simulink model "P702_NI_SoftECU"  (R2019a)
settings: Solver=ode1  StartTime=0.0  StopTime=Inf  FixedStep=0.001  RelTol=1e-3  EnableMultiTasking=on
PreLoadFcn:
  | run '.\VeriStand_BlockSet\NIVeriStandAddPaths.m'
undefined symbols (not defined in the file or in its folder): magnitude
libraries: simulink x83, simulink_extras x1
(part 62 of 76)

== system P702_NI_SoftECU/SoftECU/PCM/Logic1/Key ==
  Bus Creator1 : BusCreator  Inputs=4
  Constant : Constant
  Constant1 : Constant
  Constant2 : Constant
  Constant3 : Constant  Value=3
  Data Type Conversion : DataTypeConversion
  Data Type Conversion1 : DataTypeConversion
  Data Type Conversion2 : DataTypeConversion
  KeyPostn_No : S-Function  Priority=5  FunctionName=NIVeriStandIO  Parameters=width dtype portnum stime stype btype  SFunctionDeploymentMode=off  EnableBusSupport=off  mask(NI VeriStand Inport){portnum=5, width=-1, stime=-1, dtype=auto, stype=auto, btype=1}
      mask prompts: portnum "Port number:"; width "Port dimensions (-1 for dynamically sized):"; stime "Sample time (-1 for inherited):"; dtype "Data type:"; stype "Signal type:"; btype "Block type:"
      mask help: Use this inport on any level of nested subsystems to allow NI VeriStand software to map signals to it.
      mask init:
      | NIVeriStandIO_init;
      settings: CopyFcn=NIVeriStand_MDL_functions('', 'IO_copy');  DeleteFcn=NIVeriStand_MDL_functions('', 'IO_delete');  MoveFcn=set_param(gcb, 'Mask', 'on');
      mask Callback portnum: NIVeriStand_MDL_functions('', 'IO_setportnum');
      mask TypeOptions dtype: auto | double | single | int8 | uint8 | int16 | uint16 | int32 | uint32 | boolean
      mask Callback dtype: NIVeriStand_MDL_functions('', 'IO_booleansignal');
      mask TypeOptions stype: auto | real | complex
      mask Display:
      | patch([-x x], [-y y], [.90980 .81960 .32156]);
      | plot([xrad -x x xrad], [yrad -y y yrad]);
      | fprintf('NI In%d', portnum);
  KeyType_No : Constant
  KvActive : S-Function  Priority=1  FunctionName=NIVeriStandIO  Parameters=width dtype portnum stime stype btype  SFunctionDeploymentMode=off  EnableBusSupport=off  mask(NI VeriStand Inport){portnum=1, width=-1, stime=-1, dtype=auto, stype=auto, btype=1}
      mask prompts: portnum "Port number:"; width "Port dimensions (-1 for dynamically sized):"; stime "Sample time (-1 for inherited):"; dtype "Data type:"; stype "Signal type:"; btype "Block type:"
      mask help: Use this inport on any level of nested subsystems to allow NI VeriStand software to map signals to it.
      mask init:
      | NIVeriStandIO_init;
      settings: CopyFcn=NIVeriStand_MDL_functions('', 'IO_copy');  DeleteFcn=NIVeriStand_MDL_functions('', 'IO_delete');  MoveFcn=set_param(gcb, 'Mask', 'on');
      mask Callback portnum: NIVeriStand_MDL_functions('', 'IO_setportnum');
      mask TypeOptions dtype: auto | double | single | int8 | uint8 | int16 | uint16 | int32 | uint32 | boolean
      mask Callback dtype: NIVeriStand_MDL_functions('', 'IO_booleansignal');
      mask TypeOptions stype: auto | real | complex
      mask Display:
      | patch([-x x], [-y y], [.90980 .81960 .32156]);
      | plot([xrad -x x xrad], [yrad -y y yrad]);
      | fprintf('NI In%d', portnum);
  Logical Operator1 : Logic  Operator=OR  AllPortsSameDT=off  OutDataTypeStr=boolean
  PowerStates : Subsystem
  Start/Stop_Pulsing : Subsystem
  StartBttnPressReq_No : S-Function  Priority=3  FunctionName=NIVeriStandIO  Parameters=width dtype portnum stime stype btype  SFunctionDeploymentMode=off  EnableBusSupport=off  mask(NI VeriStand Inport){portnum=3, width=-1, stime=-1, dtype=auto, stype=auto, btype=1}
      mask prompts: portnum "Port number:"; width "Port dimensions (-1 for dynamically sized):"; stime "Sample time (-1 for inherited):"; dtype "Data type:"; stype "Signal type:"; btype "Block type:"
      mask help: Use this inport on any level of nested subsystems to allow NI VeriStand software to map signals to it.
      mask init:
      | NIVeriStandIO_init;
      settings: CopyFcn=NIVeriStand_MDL_functions('', 'IO_copy');  DeleteFcn=NIVeriStand_MDL_functions('', 'IO_delete');  MoveFcn=set_param(gcb, 'Mask', 'on');
      mask Callback portnum: NIVeriStand_MDL_functions('', 'IO_setportnum');
      mask TypeOptions dtype: auto | double | single | int8 | uint8 | int16 | uint16 | int32 | uint32 | boolean
      mask Callback dtype: NIVeriStand_MDL_functions('', 'IO_booleansignal');
      mask TypeOptions stype: auto | real | complex
      mask Display:
      | patch([-x x], [-y y], [.90980 .81960 .32156]);
      | plot([xrad -x x xrad], [yrad -y y yrad]);
      | fprintf('NI In%d', portnum);
  StartBttnSw1_B : S-Function  Priority=2  FunctionName=NIVeriStandIO  Parameters=width dtype portnum stime stype btype  SFunctionDeploymentMode=off  EnableBusSupport=off  mask(NI VeriStand Inport){portnum=2, width=-1, stime=-1, dtype=auto, stype=auto, btype=1}
      mask prompts: portnum "Port number:"; width "Port dimensions (-1 for dynamically sized):"; stime "Sample time (-1 for inherited):"; dtype "Data type:"; stype "Signal type:"; btype "Block type:"
      mask help: Use this inport on any level of nested subsystems to allow NI VeriStand software to map signals to it.
      mask init:
      | NIVeriStandIO_init;
      settings: CopyFcn=NIVeriStand_MDL_functions('', 'IO_copy');  DeleteFcn=NIVeriStand_MDL_functions('', 'IO_delete');  MoveFcn=set_param(gcb, 'Mask', 'on');
      mask Callback portnum: NIVeriStand_MDL_functions('', 'IO_setportnum');
      mask TypeOptions dtype: auto | double | single | int8 | uint8 | int16 | uint16 | int32 | uint32 | boolean
      mask Callback dtype: NIVeriStand_MDL_functions('', 'IO_booleansignal');
      mask TypeOptions stype: auto | real | complex
      mask Display:
      | patch([-x x], [-y y], [.90980 .81960 .32156]);
      | plot([xrad -x x xrad], [yrad -y y yrad]);
      | fprintf('NI In%d', portnum);
  Switch{,1..3} (4 alike) : Switch  Criteria=u2 > Threshold
  Switch_NI_Port_Pcm : S-Function  Priority=4  FunctionName=NIVeriStandIO  Parameters=width dtype portnum stime stype btype  SFunctionDeploymentMode=off  EnableBusSupport=off  mask(NI VeriStand Inport){portnum=4, width=-1, stime=-1, dtype=auto, stype=auto, btype=1}
      mask prompts: portnum "Port number:"; width "Port dimensions (-1 for dynamically sized):"; stime "Sample time (-1 for inherited):"; dtype "Data type:"; stype "Signal type:"; btype "Block type:"
      mask help: Use this inport on any level of nested subsystems to allow NI VeriStand software to map signals to it.
      mask init:
      | NIVeriStandIO_init;
      settings: CopyFcn=NIVeriStand_MDL_functions('', 'IO_copy');  DeleteFcn=NIVeriStand_MDL_functions('', 'IO_delete');  MoveFcn=set_param(gcb, 'Mask', 'on');
      mask Callback portnum: NIVeriStand_MDL_functions('', 'IO_setportnum');
      mask TypeOptions dtype: auto | double | single | int8 | uint8 | int16 | uint16 | int32 | uint32 | boolean
      mask Callback dtype: NIVeriStand_MDL_functions('', 'IO_booleansignal');
      mask TypeOptions stype: auto | real | complex
      mask Display:
      | patch([-x x], [-y y], [.90980 .81960 .32156]);
      | plot([xrad -x x xrad], [yrad -y y yrad]);
      | fprintf('NI In%d', portnum);
  Out1 : Outport
  wires:
  KeyType_No/1 -> Bus Creator1/2  "KeyType_No"
  Switch3/1 -> PowerStates/1(In1), Bus Creator1/3  "KeyPostn_No"
  Bus Creator1/1 -> Out1/1  "Key"
  PowerStates/1(Out1) -> Bus Creator1/4  "PowerStates"
  Logical Operator1/1 -> PowerStates/2(In2), Bus Creator1/1  "StartBttnSw1_B"
  Start/Stop_Pulsing/1(Out1) -> Logical Operator1/1
  StartBttnSw1_B/1 -> Data Type Conversion1/1
  StartBttnPressReq_No/1 -> Switch/1
  KvActive/1 -> Switch2/1
  Switch/1 -> Start/Stop_Pulsing/1(In1)
  Switch1/1 -> Logical Operator1/2
  Switch2/1 -> PowerStates/3(In3)
  Switch_NI_Port_Pcm/1 -> Data Type Conversion/1
  KeyPostn_No/1 -> Switch3/1
  Constant/1 -> Switch/3
  Constant1/1 -> Data Type Conversion2/1
  Constant2/1 -> Switch2/3
  Constant3/1 -> Switch3/3
  Data Type Conversion/1 -> Switch3/2, Switch2/2, Switch1/2, Switch/2
  Data Type Conversion1/1 -> Switch1/1
  Data Type Conversion2/1 -> Switch1/3

== system P702_NI_SoftECU/SoftECU/PCM/Logic1/Pedals ==
  FromMdl : Inport
  Bias : Bias  Bias=1
  BrakeLight : Constant  Value=0
  Bus Creator : BusCreator  Inputs=7
  Bus Selector : BusSelector  OutputSignals=CluBottomOfTravelSwtch_B,Throttle[percentage],BrkLightSwtch_B
  Constant : Constant  Value=3
  Derivative1 : Derivative
  Derivative2 : Derivative
  Pedals : Outport
  wires:
  Bias/1 -> Bus Creator/3  "BrakePdlDrvAppl"
  FromMdl/1 -> Bus Selector/1
  BrakeLight/1 -> Bias/1
  Derivative2/1 -> Bus Creator/2  "ApedPosRate"
  Bus Selector/2 -> Derivative2/1, Bus Creator/5  "<Throttle[percentage]>"
  Bus Creator/1 -> Pedals/1  "Pedals"
  Bus Selector/1 -> Derivative1/1, Bus Creator/4  "<CluBottomOfTravelSwtch_B>"
  Derivative1/1 -> Bus Creator/1  "CluPdlRate"
  Bus Selector/3 -> Bus Creator/6  "<BrkLightSwtch_B>"
  Constant/1 -> Bus Creator/7  "CluPdlPosPcMeas_D_Qf"

== system P702_NI_SoftECU/SoftECU/PCM/Logic1/PrplWhlTot2Calc ==
  note: R = -1
      | N = 0
      | 1 ... 6 =  1 ... 6
  note: -> Tire Torque
  Gear : Inport
  Trq_Engine [Nm] : Inport  Port=2
  GetTransmissionRatio : Subsystem
      mask Display: disp('Get current transmission ratio')
  Mult : Product  RndMeth=Zero
  PrplWhlTot_Tq : Outport
  wires:
  Gear/1 -> GetTransmissionRatio/1(Gear[-])
  GetTransmissionRatio/1(Transmission_Ratio[-]) -> Mult/2
  Trq_Engine [Nm]/1 -> Mult/1
  Mult/1 -> PrplWhlTot_Tq/1

== system P702_NI_SoftECU/SoftECU/PCM/Logic1/ReValueStates ==
  note: SelectorLever[-3T|-2P|-1R|0N|1D]
  note: GearlvrPosDActl[-1Unknown|0P|1R|2N|3D]
  GearLvr[-] : Inport
  AddOffset_for_R-N_gears : Sum
  OffsetForSw : Constant  Value=2
  Transmission_Ratio[-] : Outport
  wires:
  AddOffset_for_R-N_gears/1 -> Transmission_Ratio[-]/1  "GearLvrPos_D_ActlPart"
  OffsetForSw/1 -> AddOffset_for_R-N_gears/2
  GearLvr[-]/1 -> AddOffset_for_R-N_gears/1

== system P702_NI_SoftECU/SoftECU/PCM/Logic1/Speed_Accel_Controller ==
  note: ACC status = 0:
      | ACC off-> ignore accel and decel control, throttle and brake controlled by speed controller
      | ACC status = 1:
      | ACC ON->ignore speed controller, throttle and brake controller by acceleration controller
      | ver. 10/23/2018 ;
  ACC_Status : Inport
  Veh_Spd : Inport  Port=2
  Desired_Speed : Inport  Port=3
  vehicle_accel : Inport  Port=4
  Desried_accel : Inport  Port=5
  cmbb_rq : Inport  Port=6
  MRR : Inport  Port=7
  ACC_Accel_Controller : Subsystem
  BrakeMSPress_switch : MultiPortSwitch  DataPortOrder=Zero-based contiguous  Inputs=2  zeroidx=on
  Compare To Constant : simulink/Logic and Bit Operations/Compare To Constant  relop===  const=5  OutDataTypeStr=boolean
  Compare To Constant1 : simulink/Logic and Bit Operations/Compare To Constant  relop===  const=4  OutDataTypeStr=boolean
  Ground : Ground
  Logical Operator : Logic  Operator=OR  AllPortsSameDT=off  OutDataTypeStr=boolean
  MATLAB Function : MATLAB Function  TreatAsAtomicUnit=on
  MATLAB Function1 : MATLAB Function  TreatAsAtomicUnit=on
  Speed_Controller : Subsystem
  Terminator : Terminator
  Terminator1 : Terminator
  Terminator3 : Terminator
  throttle_switch : MultiPortSwitch  DataPortOrder=Zero-based contiguous  Inputs=2  zeroidx=on
  throttle_position : Outport
  brake_MS_pressure : Outport  Port=2
  wires:
  Speed_Controller/1(Throttle_Pos) -> MATLAB Function1/1(throttle_pos)
  ACC_Accel_Controller/1(Throttle_Pos) -> throttle_switch/3
  Speed_Controller/2(Brake_MS_Pressure) -> BrakeMSPress_switch/2
  ACC_Accel_Controller/2(Brake_MS_Pressure) -> BrakeMSPress_switch/3
  ACC_Status/1 -> Compare To Constant1/1, Compare To Constant/1
  Veh_Spd/1 -> Terminator/1, Speed_Controller/1(Veh_Spd)
  throttle_switch/1 -> throttle_position/1
  vehicle_accel/1 -> ACC_Accel_Controller/1(Vehicle_Ax)
  Desried_accel/1 -> ACC_Accel_Controller/2(Desried_accel)
  Logical Operator/1 -> BrakeMSPress_switch/1, throttle_switch/1
  BrakeMSPress_switch/1 -> brake_MS_pressure/1
  Compare To Constant/1 -> Logical Operator/1
  Compare To Constant1/1 -> Logical Operator/2
  cmbb_rq/1 -> MATLAB Function1/2(cmbb_req)
  MRR/1 -> Terminator1/1
  Ground/1 -> MATLAB Function/4(mrr), MATLAB Function/3(desired_speed_rq), MATLAB Function/2(cmbb_req), MATLAB Function/1(veh_speed)
  MATLAB Function/1(desired_speed) -> Terminator3/1
  Desired_Speed/1 -> Speed_Controller/2(Desried_Spd)
  MATLAB Function1/1(throttle) -> throttle_switch/2

== system P702_NI_SoftECU/SoftECU/PCM/Logic1/StartStop ==
  Eng_D_Stat : Inport
  Cranking_status : Inport  Port=2
  Compare To Constant : simulink/Logic and Bit Operations/Compare To Constant  relop===  const=1  OutDataTypeStr=uint8
  Logical Operator : Logic  Operator=NOT  AllPortsSameDT=off  OutDataTypeStr=boolean
  Logical Operator1 : Logic  AllPortsSameDT=off  OutDataTypeStr=boolean
  dt_ElPw_D_StatStrtStop : DataTypeConversion  RndMeth=Zero
  StatStrtStop : Outport
  Cranking_status_out : Outport  Port=2
  wires:
  Logical Operator1/1 -> dt_ElPw_D_StatStrtStop/1
  Logical Operator/1 -> Logical Operator1/2
  Compare To Constant/1 -> Logical Operator1/1
  Cranking_status/1 -> Cranking_status_out/1, Logical Operator/1  "PcmCrankingStatus_B"
  dt_ElPw_D_StatStrtStop/1 -> StatStrtStop/1  "StatStrtStop"
  Eng_D_Stat/1 -> Compare To Constant/1  "Eng_D_Stat_No"

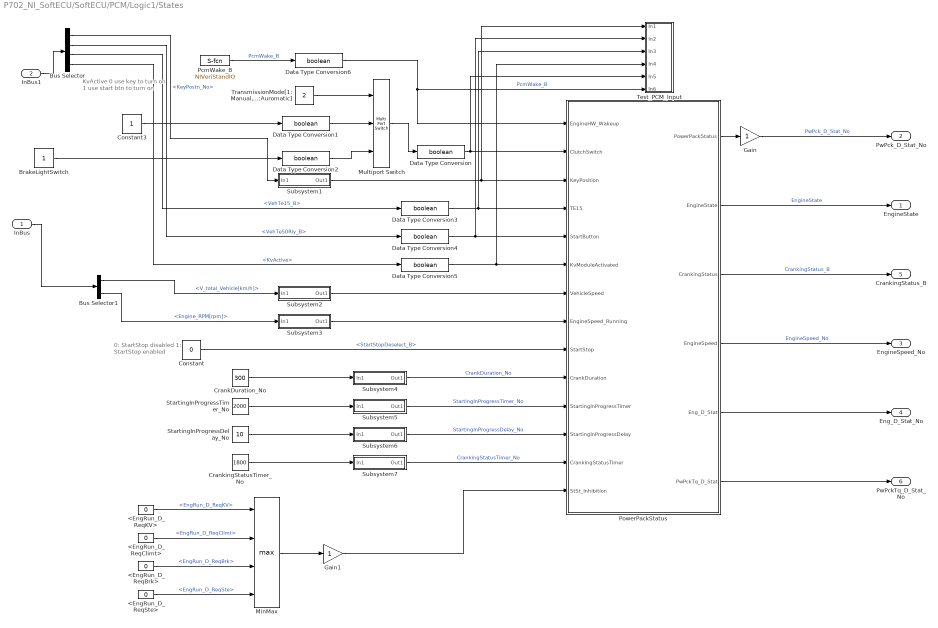
== system P702_NI_SoftECU/SoftECU/PCM/Logic1/States ==
  note: KvActive
      | 0 use key to turn on
      | 1 use start btn to turn on
  note: 0: StartStop disabled
      | 1:  StartStop enabled
  InBus : Inport
  InBus1 : Inport  Port=2
  <EngRun_D_ReqBrk> : Constant  Value=0  OutDataTypeStr=double
  <EngRun_D_ReqClimt> : Constant  Value=0  OutDataTypeStr=double
  <EngRun_D_ReqKV> : Constant  Value=0  OutDataTypeStr=double
  <EngRun_D_ReqSte> : Constant  Value=0  OutDataTypeStr=double
  BrakeLightSwitch : Constant
  Bus Selector : BusSelector  OutputSignals=KeyPostn_No,PowerStates.VehTe50Rly_B,PowerStates.VehTe15_B,PowerStates.KvActive
  Bus Selector1 : BusSelector  OutputSignals=V_total_Vehicle[km/h],Engine_RPM[rpm]
  Constant : Constant  Value=0
  Constant3 : Constant
  CrankDuration_No : Constant  Value=300
  CrankingStatusTimer_No : Constant  Value=1800
  Data Type Conversion{,1..6} (7 alike) : DataTypeConversion  OutDataTypeStr=boolean
  Gain : Gain
  Gain1 : Gain
  MinMax : MinMax  Function=max  Inputs=4
  Multiport Switch : MultiPortSwitch  Inputs=2
  PcmWake_B : S-Function  Priority=1  FunctionName=NIVeriStandIO  Parameters=width dtype portnum stime stype btype  SFunctionDeploymentMode=off  EnableBusSupport=off  mask(NI VeriStand Inport){portnum=1, width=-1, stime=-1, dtype=auto, stype=auto, btype=1}
      mask prompts: portnum "Port number:"; width "Port dimensions (-1 for dynamically sized):"; stime "Sample time (-1 for inherited):"; dtype "Data type:"; stype "Signal type:"; btype "Block type:"
      mask help: Use this inport on any level of nested subsystems to allow NI VeriStand software to map signals to it.
      mask init:
      | NIVeriStandIO_init;
      settings: CopyFcn=NIVeriStand_MDL_functions('', 'IO_copy');  DeleteFcn=NIVeriStand_MDL_functions('', 'IO_delete');  MoveFcn=set_param(gcb, 'Mask', 'on');
      mask Callback portnum: NIVeriStand_MDL_functions('', 'IO_setportnum');
      mask TypeOptions dtype: auto | double | single | int8 | uint8 | int16 | uint16 | int32 | uint32 | boolean
      mask Callback dtype: NIVeriStand_MDL_functions('', 'IO_booleansignal');
      mask TypeOptions stype: auto | real | complex
      mask Display:
      | patch([-x x], [-y y], [.90980 .81960 .32156]);
      | plot([xrad -x x xrad], [yrad -y y yrad]);
      | fprintf('NI In%d', portnum);
  PowerPackStatus : Stateflow chart  TreatAsAtomicUnit=on
  StartingInProgressDelay_No : Constant  Value=10
  StartingInProgressTimer_No : Constant  Value=2000
  Subsystem1 : Subsystem
  Subsystem2 : Subsystem
  Subsystem3 : Subsystem
  Subsystem4 : Subsystem
  Subsystem5 : Subsystem
  Subsystem6 : Subsystem
  Subsystem7 : Subsystem
  Test_PCM_Input : Subsystem
  TransmissionMode[1:Manual,2:Auromatic] : Constant  Value=2
  EngineState : Outport
  "PwPck_D_Stat_No " : Outport  Port=2
  EngineSpeed_No : Outport  Port=3
  Eng_D_Stat_No : Outport  Port=4
  CrankingStatus_B : Outport  Port=5
  PwPckTq_D_Stat_No : Outport  Port=6
  wires:
  CrankingStatusTimer_No/1 -> Subsystem7/1(In1)
  StartingInProgressDelay_No/1 -> Subsystem6/1(In1)
  StartingInProgressTimer_No/1 -> Subsystem5/1(In1)
  CrankDuration_No/1 -> Subsystem4/1(In1)
  Bus Selector/3 -> Data Type Conversion3/1  "<VehTe15_B>"
  Bus Selector/1 -> Subsystem1/1(In1)  "<KeyPostn_No>"
  Bus Selector/2 -> Data Type Conversion4/1  "<VehTe50Rly_B>"
  Gain1/1 -> PowerPackStatus/14(StSt_Inhibition)
  PcmWake_B/1 -> Data Type Conversion6/1  "PcmWake_B"
  Subsystem7/1(Out1) -> PowerPackStatus/13(CrankingStatusTimer)  "CrankingStatusTimer_No"
  Subsystem6/1(Out1) -> PowerPackStatus/12(StartingInProgressDelay)  "StartingInProgressDelay_No"
  Subsystem5/1(Out1) -> PowerPackStatus/11(StartingInProgressTimer)  "StartingInProgressTimer_No"
  Subsystem4/1(Out1) -> PowerPackStatus/10(CrankDuration)  "CrankDuration_No"
  Subsystem3/1(Out1) -> PowerPackStatus/8(EngineSpeed_Running)
  Subsystem2/1(Out1) -> PowerPackStatus/7(VehicleSpeed)
  Subsystem1/1(Out1) -> Test_PCM_Input/1(In1), PowerPackStatus/3(KeyPosition)
  Data Type Conversion5/1 -> Test_PCM_Input/4(In4), PowerPackStatus/6(KvModuleActivated)
  Data Type Conversion4/1 -> Test_PCM_Input/2(In2), PowerPackStatus/5(StartButton)
  Data Type Conversion3/1 -> Test_PCM_Input/3(In3), PowerPackStatus/4(TE15)
  TransmissionMode[1:Manual,2:Auromatic]/1 -> Multiport Switch/1
  Bus Selector1/2 -> Subsystem3/1(In1)  "<Engine_RPM[rpm]>"
  PowerPackStatus/6(PwPckTq_D_Stat) -> PwPckTq_D_Stat_No/1
  PowerPackStatus/5(Eng_D_Stat) -> Eng_D_Stat_No/1
  Data Type Conversion2/1 -> Multiport Switch/3
  Data Type Conversion1/1 -> Multiport Switch/2
  Data Type Conversion/1 -> Test_PCM_Input/5(In5), PowerPackStatus/2(ClutchSwitch)
  BrakeLightSwitch/1 -> Data Type Conversion2/1
  Constant3/1 -> Data Type Conversion1/1
  Multiport Switch/1 -> Data Type Conversion/1
  MinMax/1 -> Gain1/1
  PowerPackStatus/4(EngineSpeed) -> EngineSpeed_No/1  "EngineSpeed_No"
  PowerPackStatus/3(CrankingStatus) -> CrankingStatus_B/1  "CrankingStatus_B"
  Constant/1 -> PowerPackStatus/9(StartStop)  "<StartStopDeselect_B>"
  Bus Selector1/1 -> Subsystem2/1(In1)  "<V_total_Vehicle[km/h]>"
  PowerPackStatus/2(EngineState) -> EngineState/1  "EngineState"
  PowerPackStatus/1(PowerPackStatus) -> Gain/1
  Gain/1 -> "PwPck_D_Stat_No "/1  "PwPck_D_Stat_No"
  InBus1/1 -> Bus Selector/1
  InBus/1 -> Bus Selector1/1
  Bus Selector/4 -> Data Type Conversion5/1  "<KvActive>"
  <EngRun_D_ReqClimt>/1 -> MinMax/2  "<EngRun_D_ReqClimt>"
  <EngRun_D_ReqKV>/1 -> MinMax/1  "<EngRun_D_ReqKV>"
  <EngRun_D_ReqBrk>/1 -> MinMax/3  "<EngRun_D_ReqBrk>"
  <EngRun_D_ReqSte>/1 -> MinMax/4  "<EngRun_D_ReqSte>"
  Data Type Conversion6/1 -> Test_PCM_Input/6(In6), PowerPackStatus/1(EngineHW_Wakeup)  "PcmWake_B"

== system P702_NI_SoftECU/SoftECU/PCM/Mapping/EngBrakeData ==
  note: Where to map this Brake Switch Signal ??
  In1 : Inport
  Bus Creator1 : BusCreator  Inputs=2
  Bus Selector : BusSelector  OutputSignals=Pedals.BrkLightSwtch_B,Pedals.BrakePdlDrvAppl
  Gain : Gain
  Gain1 : Gain
  Out1 : Outport
  wires:
  In1/1 -> Bus Selector/1
  Bus Creator1/1 -> Out1/1  "EngBrakeData"
  Gain1/1 -> Bus Creator1/2  "BpedDrvAppl_D_Actl"
  Gain/1 -> Bus Creator1/1  "BrkOnOffSwtch_D_Actl"
  Bus Selector/2 -> Gain1/1  "<BrakePdlDrvAppl>"
  Bus Selector/1 -> Gain/1  "<BrkLightSwtch_B>"

== system P702_NI_SoftECU/SoftECU/PCM/Mapping/EngVehicleSpThrottle ==
  In1 : Inport
  Bus Creator1 : BusCreator  Inputs=5
  Bus Selector : BusSelector  OutputSignals=EngVehSpeed.VehicleSpeed_No,Pedals.Throttle[percentage],Pedals.ApedPosRate,ApedPosPcActl_No_Cs,ApedPos_Pc_ActlArb_No_Cnt
  Gain{,1..4} (5 alike) : Gain
  Out1 : Outport
  wires:
  Gain2/1 -> Bus Creator1/3  "ApedPos_PcRate_ActlArb"
  Bus Selector/3 -> Gain2/1  "<ApedPosRate>"
  Bus Selector/1 -> Gain/1  "<VehicleSpeed_No>"
  Gain/1 -> Bus Creator1/1  "EngAout_N_Actl"
  Bus Creator1/1 -> Out1/1  "EngVehicleSpThrottle"
  In1/1 -> Bus Selector/1
  Bus Selector/2 -> Gain1/1  "<Throttle[percentage]>"
  Gain1/1 -> Bus Creator1/2  "ApedPos_Pc_ActlArb"
  Bus Selector/4 -> Gain3/1  "<ApedPosPcActl_No_Cs>"
  Gain3/1 -> Bus Creator1/4  "ApedPosPcActl_No_Cs"
  Bus Selector/5 -> Gain4/1  "<ApedPos_Pc_ActlArb_No_Cnt>"
  Gain4/1 -> Bus Creator1/5  "ApedPos_Pc_ActlArb_No_Cnt"

== system P702_NI_SoftECU/SoftECU/PCM/Mapping/EngVehicleSpThrottle2 ==
  In1 : Inport
  Bus Creator1 : BusCreator  Inputs=3
  Bus Selector : BusSelector  OutputSignals=EngVehSpeed.VehicleSpeed_No,EngVehSpeed.CalcGearRvrseActv,EngVehSpeed.Veh_V_RqCcSet
  Gain : Gain
  Gain1 : Gain
  Gain2 : Gain
  Out1 : Outport
  wires:
  Gain2/1 -> Bus Creator1/3  "Veh_V_RqCcSet"
  Bus Selector/3 -> Gain2/1  "<Veh_V_RqCcSet>"
  Gain1/1 -> Bus Creator1/2  "GearRvrse_D_Actl"
  Bus Selector/2 -> Gain1/1  "<CalcGearRvrseActv>"
  In1/1 -> Bus Selector/1
  Bus Creator1/1 -> Out1/1  "EngVehicleSpThrottle2"
  Gain/1 -> Bus Creator1/1  "Veh_V_ActlEng"
  Bus Selector/1 -> Gain/1  "<VehicleSpeed_No>"

== system P702_NI_SoftECU/SoftECU/PCM/Mapping/EngineClimateData ==
  In1 : Inport
  Bus Creator1 : BusCreator  Inputs=3
  Bus Selector : BusSelector  OutputSignals=EngineAcc_No
  Constant : Constant  Value=20
  Gain : Gain
  Gain1 : Gain
  Gain2 : Gain
  Out1 : Outport
  wires:
  Constant/1 -> Gain1/1, Gain2/1  "<AmbientAirTemp_No>"
  Gain2/1 -> Bus Creator1/3  "AirAmb_Te_ActlFilt"
  Gain1/1 -> Bus Creator1/2  "AirAmb_Te_Actl"
  Bus Selector/1 -> Gain/1  "<EngineAcc_No>"
  Gain/1 -> Bus Creator1/1  "EngAout_Aa_Actl"
  Bus Creator1/1 -> Out1/1  "EngineClimateData"
  In1/1 -> Bus Selector/1

== system P702_NI_SoftECU/SoftECU/PCM/Mapping/EngineClutchData ==
  In1 : Inport
  Bus Creator1 : BusCreator  Inputs=3
  Bus Selector : BusSelector  OutputSignals=Pedals.CluPdlRate,Pedals.CluBottomOfTravelSwtch_B,Pedals.CluPdlPosPcMeas_D_Qf
  Gain : Gain
  Gain1 : Gain
  Out1 : Outport
  wires:
  Gain1/1 -> Bus Creator1/2  "CluPdlPos_Pc_Meas"
  Bus Selector/2 -> Gain1/1  "<CluBottomOfTravelSwtch_B>"
  In1/1 -> Bus Selector/1
  Bus Creator1/1 -> Out1/1  "Engine_Clutch_Data"
  Gain/1 -> Bus Creator1/1  "CluPdl_PcRate_Actl"
  Bus Selector/1 -> Gain/1  "<CluPdlRate>"
  Bus Selector/3 -> Bus Creator1/3  "<CluPdlPosPcMeas_D_Qf>"

== system P702_NI_SoftECU/SoftECU/PCM/Mapping/EngineData_7 ==
  note: Connect Signals
  note: Vehicle_Speed
  note: RX-Status of EngineData_7 on HS1CAN
  In1 : Inport
  Bus Creator : BusCreator  Inputs=2
  Constant_1 : Constant  Value=0
  Constant_2 : Constant  Value=0
  Constant_3 : Constant  Value=0
  Count : Subsystem
  Count1 : Subsystem
  FuelFlw_Vl_Dsply : Subsystem
  FuelFlw_Vl_DsplyCanSignal_No : Terminator
  FuelFlw_Vl_DsplyElapsedTime_No : Terminator
  FuelFlw_Vl_DsplyNoCountSet_No : Constant
  FuelFlw_Vl_DsplyNumOfPeriods_No : Terminator
  FuelFlw_Vl_DsplyOverAllCount_No : Terminator
  FuelFlw_Vl_DsplyStepSize_No : Terminator
  Max_Value_FuelFlw_Vl_Dsply : Constant  Value=1024
  Max_Value_OdoCount : Constant  Value=255
  Memory : Memory
  ODoCount : Subsystem
  OdoCountCanSignal_No : Terminator
  OdoCountElapsedTime_No : Terminator
  OdoCountEnable_B : Constant
  OdoCountMsgCycleTime : Constant
  OdoCountNumOfPeriods_No : Terminator
  OdoCountOverAllCount_No : Terminator
  OdoCountRunTime_No : Constant
  OdoCountStepSize_No : Terminator
  OdoCountStimuSw_B : Constant
  OdoNoCountSet_No : Constant
  Rounding Function1 : Rounding
  Scale : Gain  Gain=0.2
  Scale1 : Gain  Gain=25
  Scale2 : Gain  Gain=0.2
  Scale3 : Gain  Gain=25
  Switch : Switch  Criteria=u2 ~= 0
  Switch1 : Switch  Criteria=u2 ~= 0
  Terminator : Terminator
  Terminator1 : Terminator
  Terminator_3 : Terminator
  scaling : Subsystem
  scaling_ : Subsystem
  Out1 : Outport
  wires:
  In1/1 -> Terminator_3/1
  Rounding Function1/1 -> Switch/3
  Count1/2(OverallCount) -> Terminator1/1
  Count/2(OverallCount) -> Terminator/1
  scaling_/1(Out1) -> Count1/1(Stepsize)
  FuelFlw_Vl_Dsply/4(ElapsedTime) -> FuelFlw_Vl_DsplyElapsedTime_No/1
  FuelFlw_Vl_Dsply/5(NumPeriods) -> FuelFlw_Vl_DsplyNumOfPeriods_No/1
  FuelFlw_Vl_Dsply/3(OverallCount) -> FuelFlw_Vl_DsplyOverAllCount_No/1
  Scale3/1 -> FuelFlw_Vl_DsplyCanSignal_No/1
  Scale2/1 -> OdoCountCanSignal_No/1
  FuelFlw_Vl_Dsply/1(StepSize) -> FuelFlw_Vl_DsplyStepSize_No/1
  Switch1/1 -> Scale1/1
  FuelFlw_Vl_Dsply/2(CAN_signal) -> Scale3/1, Switch1/1
  FuelFlw_Vl_DsplyNoCountSet_No/1 -> FuelFlw_Vl_Dsply/4(NumberOfCounts)
  Scale1/1 -> Bus Creator/2  "FuelFlw_Vl_Dsply"
  Scale/1 -> Bus Creator/1  "OdoCount"
  ODoCount/5(NumPeriods) -> OdoCountNumOfPeriods_No/1
  ODoCount/4(ElapsedTime) -> OdoCountElapsedTime_No/1
  ODoCount/3(OverallCount) -> OdoCountOverAllCount_No/1
  ODoCount/1(StepSize) -> OdoCountStepSize_No/1
  OdoCountMsgCycleTime/1 -> FuelFlw_Vl_Dsply/3(MsgCycleTime), ODoCount/3(MsgCycleTime)
  ODoCount/2(CAN_signal) -> Scale2/1, Switch/1
  OdoCountRunTime_No/1 -> FuelFlw_Vl_Dsply/5(Runtime), ODoCount/5(Runtime)
  OdoNoCountSet_No/1 -> ODoCount/4(NumberOfCounts)
  OdoCountEnable_B/1 -> FuelFlw_Vl_Dsply/1(Enable), ODoCount/1(Enable)
  Memory/1 -> ODoCount/2(Trigger), Count/Enable, FuelFlw_Vl_Dsply/2(Trigger), Count1/Enable
  scaling/1(Out1) -> Count/1(Stepsize)
  Switch/1 -> Scale/1  "OdoCount"
  OdoCountStimuSw_B/1 -> Switch1/2, Switch/2  "OdoCountStimu_Sw_B"
  Constant_2/1 -> scaling/1(In1)  "v_x_Vehicle_CoG[km|h]"
  Constant_3/1 -> Count/3(Reset), FuelFlw_Vl_Dsply/6(Reset), Count1/3(Reset), ODoCount/6(Reset)  "VehTe15_B"
  Constant_1/1 -> Memory/1  "RX_Status"
  Max_Value_FuelFlw_Vl_Dsply/1 -> Count1/2(MaxValue)
  Max_Value_OdoCount/1 -> Count/2(MaxValue)
  Count1/1(OdoCount) -> Switch1/3  "FuelFlw_Vl_Dsply"
  Count/1(OdoCount) -> Rounding Function1/1  "OdoCount"
  Bus Creator/1 -> Out1/1  "EngineData_7"

== system P702_NI_SoftECU/SoftECU/PCM/Mapping/PowertrainData_10 ==
  In1 : Inport
  Bus Creator1 : BusCreator  Inputs=3
  Bus Selector : BusSelector  OutputSignals=GearPos_No_Cs,GearPos_No_Cnt,GearLvr_D_ActlDrv
  Gain : Gain
  Gain1 : Gain
  Gain2 : Gain
  Out1 : Outport
  wires:
  Gain1/1 -> Bus Creator1/2  "GearPos_No_Cnt"
  Bus Selector/2 -> Gain1/1  "<GearPos_No_Cnt>"
  In1/1 -> Bus Selector/1
  Bus Creator1/1 -> Out1/1  "PowertrainData_10"
  Gain/1 -> Bus Creator1/1  "GearPos_No_Cs"
  Bus Selector/1 -> Gain/1  "<GearPos_No_Cs>"
  Bus Selector/3 -> Gain2/1  "<GearLvr_D_ActlDrv>"
  Gain2/1 -> Bus Creator1/3  "GearLvr_D_ActlDrv"

== system P702_NI_SoftECU/SoftECU/PCM/Mapping/TorqueDataEngFlags ==
  note: PwPckTq_D_Stat
      | -------------------------------------------
      | 0        PwPckOff_TqNotAvailable
      |  1         PwPckOn_TqNotAvailable
      | 2          StartInPrgrss_TqNotAvail
      |  3              PwPckOn_TqAvailable
  note: GGEA1.3 LC:
      |
      | Eng_D_Stat
      | --------------------------------
      | 0                       EngOff
      | 1                       EngOn
      | 2       EngAutoStopped
      | 3                      n. used
  note: CGEA1.1:
      |
      | EngineState
      | ----------------------
      | 0                Off
      | 1          Ready
      | 2     Cranking
      | 3      Running
      | 4         Stalled
      | 5       Afterrun
      | 6   Shutdown
      | 7            n.def.
  In1 : Inport
  Bus Creator1 : BusCreator  Inputs=3
  Bus Selector : BusSelector  OutputSignals=PrplWhlTot_Tq_Rq,PrplWhlTotTqRq_No_Cs,PrplWhlTot_Tq_Rq_No_Cnt
  Gain : Gain
  Gain1 : Gain
  Gain2 : Gain
  Out1 : Outport
  wires:
  In1/1 -> Bus Selector/1
  Bus Creator1/1 -> Out1/1  "VehicleOperatingModes"
  Bus Selector/1 -> Gain/1  "<PrplWhlTot_Tq_Rq>"
  Gain/1 -> Bus Creator1/1  "PrplWhlTot_Tq_Rq"
  Gain1/1 -> Bus Creator1/2  "PrplWhlTotTqRq_No_Cs"
  Gain2/1 -> Bus Creator1/3  "PrplWhlTot_Tq_Rq_No_Cnt"
  Bus Selector/2 -> Gain1/1  "<PrplWhlTotTqRq_No_Cs>"
  Bus Selector/3 -> Gain2/1  "<PrplWhlTot_Tq_Rq_No_Cnt>"

== system P702_NI_SoftECU/SoftECU/PCM/Mapping/VehicleOperatingModes ==
  note: CGEA1.1:
      |
      | EngineState
      | ----------------------
      | 0                Off
      | 1          Ready
      | 2     Cranking
      | 3      Running
      | 4         Stalled
      | 5       Afterrun
      | 6   Shutdown
      | 7            n.def.
  note: GGEA1.3 LC:
      |
      | Eng_D_Stat
      | --------------------------------
      | 0                       EngOff
      | 1                       EngOn
      | 2       EngAutoStopped
      | 3                      n. used
  note: PwPckTq_D_Stat
      | -------------------------------------------
      | 0        PwPckOff_TqNotAvailable
      |  1         PwPckOn_TqNotAvailable
      | 2          StartInPrgrss_TqNotAvail
      |  3              PwPckOn_TqAvailable
  In1 : Inport
  Bus Creator1 : BusCreator  Inputs=5
  Bus Selector : BusSelector  OutputSignals=Eng_D_Stat_No,PwPckTq_D_Stat_No,PrplWhlTot_Tq_Rq,StartStrtStop
  Gain{,1..4} (5 alike) : Gain
  Out1 : Outport
  wires:
  Gain2/1 -> Bus Creator1/3  "PrplWhlTot2_Tq_Rq"
  Bus Selector/3 -> Gain2/1  "<PrplWhlTot_Tq_Rq>"
  Gain4/1 -> Bus Creator1/5  "ElPw_D_Stat"
  Gain3/1 -> Bus Creator1/4  "ElPw_D_StatStrtStop"
  Bus Selector/4 -> Gain3/1, Gain4/1  "<StartStrtStop>"
  Bus Selector/1 -> Gain/1  "<Eng_D_Stat_No>"
  Gain/1 -> Bus Creator1/1  "Eng_D_Stat"
  Bus Creator1/1 -> Out1/1  "VehicleOperatingModes"
  In1/1 -> Bus Selector/1
  Bus Selector/2 -> Gain1/1  "<PwPckTq_D_Stat_No>"
  Gain1/1 -> Bus Creator1/2  "PwPckTq_D_Stat"

== system P702_NI_SoftECU/SoftECU/PSCM/Logic/Checksums ==
  StePinAng_Counter : Inport
  StePinRelInit_Sns : Inport  Port=2
  StePinComp_Est : Inport  Port=3
  StePinRelCalib_Sns : Inport  Port=4
  MATLAB Function : MATLAB Function  TreatAsAtomicUnit=on
  StePw_Rq : Constant
  Out1 : Outport
  wires:
  StePinComp_Est/1 -> MATLAB Function/2(SteWhlOSRelInit2An_Est)
  StePinAng_Counter/1 -> MATLAB Function/3(SteWhlAn_No_Cnt)
  StePinRelInit_Sns/1 -> MATLAB Function/1(SteWhlRelInit2_An_Sns)
  MATLAB Function/1(CD4_SteeringAngleCS) -> Out1/1  "Checksums"
  StePw_Rq/1 -> MATLAB Function/5(StePw_Rq)
  StePinRelCalib_Sns/1 -> MATLAB Function/4(SteWhlRelCalib_An_Sns)

== system P702_NI_SoftECU/SoftECU/PSCM/Logic/Counters ==
  Counter Limited : simulink/Sources/Counter Limited  uplimit=15  tsamp=0.01
  Data Type Conversion : DataTypeConversion  OutDataTypeStr=uint8
  Out1 : Outport
  wires:
  Counter Limited/1 -> Data Type Conversion/1
  Data Type Conversion/1 -> Out1/1  "SteWhlAngleCounter"

== system P702_NI_SoftECU/SoftECU/PSCM/Logic/UnitConversion ==
  In1 : Inport
  Data Type Conversion : DataTypeConversion
  busselector2 : BusSelector  OutputSignals=Agnle_SteeringWheel[deg]
  Out1 : Outport
  wires:
  busselector2/1 -> Data Type Conversion/1  "<Agnle_SteeringWheel[deg]>"
  In1/1 -> busselector2/1
  Data Type Conversion/1 -> Out1/1  "UnitConversion"

== system P702_NI_SoftECU/SoftECU/PSCM/Mapping/SteeringPinion_Data ==
  note: Note:
      | Use Unit Conversion signal instead of steering wheel position
      |
      | Han LIU 04252017
  In1 : Inport
  Constant1 : Constant  Value=0
  Constant2 : Constant  Value=3
  Data Type Conversion{,1..3} (4 alike) : DataTypeConversion
  buscreator : BusCreator  Inputs=6
  busselector : BusSelector  OutputSignals=UnitConversion,SteWhlAngleCounter,Checksums
  Out1 : Outport
  wires:
  In1/1 -> busselector/1
  buscreator/1 -> Out1/1  "SteeringPinion_Data"
  Data Type Conversion/1 -> buscreator/1  "Angle_SteeringWheel"
  Data Type Conversion1/1 -> buscreator/2  "SteWhlAngCounter"
  Data Type Conversion2/1 -> buscreator/3  "WhlAngleCs"
  busselector/3 -> Data Type Conversion2/1  "<Checksums>"
  busselector/1 -> Data Type Conversion3/1, Data Type Conversion/1  "<UnitConversion>"
  busselector/2 -> Data Type Conversion1/1  "<SteWhlAngleCounter>"
  Data Type Conversion3/1 -> buscreator/4  "StePinRelInit_An_Sns"
  Constant1/1 -> buscreator/5  "StePw_B_Rq"
  Constant2/1 -> buscreator/6  "StePinCompAnEst_D_Qf"

== system P702_NI_SoftECU/SoftECU/RCM/Logic/Checksums ==
  Counter : Inport
  Accel_Counter : Inport  Port=2
  RollRate : Inport  Port=3
  YawRate : Inport  Port=4
  LatAccel : Inport  Port=5
  LongAccel : Inport  Port=6
  VertAccel : Inport  Port=7
  Bus Creator : BusCreator  Inputs=7
  Data Type Conversion{,1..6,10..11} (9 alike) : DataTypeConversion
  MATLAB Function : MATLAB Function  TreatAsAtomicUnit=on
  MATLAB Function1 : MATLAB Function  TreatAsAtomicUnit=on
  Rate Transition{,1..4} (5 alike) : RateTransition
  VehLat_Qf : S-Function  Priority=3  FunctionName=NIVeriStandIO  Parameters=width dtype portnum stime stype btype  SFunctionDeploymentMode=off  EnableBusSupport=off  mask(NI VeriStand Inport){portnum=3, width=-1, stime=-1, dtype=auto, stype=auto, btype=1}
      mask prompts: portnum "Port number:"; width "Port dimensions (-1 for dynamically sized):"; stime "Sample time (-1 for inherited):"; dtype "Data type:"; stype "Signal type:"; btype "Block type:"
      mask help: Use this inport on any level of nested subsystems to allow NI VeriStand software to map signals to it.
      mask init:
      | NIVeriStandIO_init;
      settings: CopyFcn=NIVeriStand_MDL_functions('', 'IO_copy');  DeleteFcn=NIVeriStand_MDL_functions('', 'IO_delete');  MoveFcn=set_param(gcb, 'Mask', 'on');
      mask Callback portnum: NIVeriStand_MDL_functions('', 'IO_setportnum');
      mask TypeOptions dtype: auto | double | single | int8 | uint8 | int16 | uint16 | int32 | uint32 | boolean
      mask Callback dtype: NIVeriStand_MDL_functions('', 'IO_booleansignal');
      mask TypeOptions stype: auto | real | complex
      mask Display:
      | patch([-x x], [-y y], [.90980 .81960 .32156]);
      | plot([xrad -x x xrad], [yrad -y y yrad]);
      | fprintf('NI In%d', portnum);
  VehLong_Qf : S-Function  Priority=4  FunctionName=NIVeriStandIO  Parameters=width dtype portnum stime stype btype  SFunctionDeploymentMode=off  EnableBusSupport=off  mask(NI VeriStand Inport){portnum=4, width=-1, stime=-1, dtype=auto, stype=auto, btype=1}
      mask prompts: portnum "Port number:"; width "Port dimensions (-1 for dynamically sized):"; stime "Sample time (-1 for inherited):"; dtype "Data type:"; stype "Signal type:"; btype "Block type:"
      mask help: Use this inport on any level of nested subsystems to allow NI VeriStand software to map signals to it.
      mask init:
      | NIVeriStandIO_init;
      settings: CopyFcn=NIVeriStand_MDL_functions('', 'IO_copy');  DeleteFcn=NIVeriStand_MDL_functions('', 'IO_delete');  MoveFcn=set_param(gcb, 'Mask', 'on');
      mask Callback portnum: NIVeriStand_MDL_functions('', 'IO_setportnum');
      mask TypeOptions dtype: auto | double | single | int8 | uint8 | int16 | uint16 | int32 | uint32 | boolean
      mask Callback dtype: NIVeriStand_MDL_functions('', 'IO_booleansignal');
      mask TypeOptions stype: auto | real | complex
      mask Display:
      | patch([-x x], [-y y], [.90980 .81960 .32156]);
      | plot([xrad -x x xrad], [yrad -y y yrad]);
      | fprintf('NI In%d', portnum);
  VehRol_Qf : S-Function  Priority=1  FunctionName=NIVeriStandIO  Parameters=width dtype portnum stime stype btype  SFunctionDeploymentMode=off  EnableBusSupport=off  mask(NI VeriStand Inport){portnum=1, width=-1, stime=-1, dtype=auto, stype=auto, btype=1}
      mask prompts: portnum "Port number:"; width "Port dimensions (-1 for dynamically sized):"; stime "Sample time (-1 for inherited):"; dtype "Data type:"; stype "Signal type:"; btype "Block type:"
      mask help: Use this inport on any level of nested subsystems to allow NI VeriStand software to map signals to it.
      mask init:
      | NIVeriStandIO_init;
      settings: CopyFcn=NIVeriStand_MDL_functions('', 'IO_copy');  DeleteFcn=NIVeriStand_MDL_functions('', 'IO_delete');  MoveFcn=set_param(gcb, 'Mask', 'on');
      mask Callback portnum: NIVeriStand_MDL_functions('', 'IO_setportnum');
      mask TypeOptions dtype: auto | double | single | int8 | uint8 | int16 | uint16 | int32 | uint32 | boolean
      mask Callback dtype: NIVeriStand_MDL_functions('', 'IO_booleansignal');
      mask TypeOptions stype: auto | real | complex
      mask Display:
      | patch([-x x], [-y y], [.90980 .81960 .32156]);
      | plot([xrad -x x xrad], [yrad -y y yrad]);
      | fprintf('NI In%d', portnum);
  VehVert_Qf : S-Function  Priority=5  FunctionName=NIVeriStandIO  Parameters=width dtype portnum stime stype btype  SFunctionDeploymentMode=off  EnableBusSupport=off  mask(NI VeriStand Inport){portnum=5, width=-1, stime=-1, dtype=auto, stype=auto, btype=1}
      mask prompts: portnum "Port number:"; width "Port dimensions (-1 for dynamically sized):"; stime "Sample time (-1 for inherited):"; dtype "Data type:"; stype "Signal type:"; btype "Block type:"
      mask help: Use this inport on any level of nested subsystems to allow NI VeriStand software to map signals to it.
      mask init:
      | NIVeriStandIO_init;
      settings: CopyFcn=NIVeriStand_MDL_functions('', 'IO_copy');  DeleteFcn=NIVeriStand_MDL_functions('', 'IO_delete');  MoveFcn=set_param(gcb, 'Mask', 'on');
      mask Callback portnum: NIVeriStand_MDL_functions('', 'IO_setportnum');
      mask TypeOptions dtype: auto | double | single | int8 | uint8 | int16 | uint16 | int32 | uint32 | boolean
      mask Callback dtype: NIVeriStand_MDL_functions('', 'IO_booleansignal');
      mask TypeOptions stype: auto | real | complex
      mask Display:
      | patch([-x x], [-y y], [.90980 .81960 .32156]);
      | plot([xrad -x x xrad], [yrad -y y yrad]);
      | fprintf('NI In%d', portnum);
  VehYaw_Qf : S-Function  Priority=2  FunctionName=NIVeriStandIO  Parameters=width dtype portnum stime stype btype  SFunctionDeploymentMode=off  EnableBusSupport=off  mask(NI VeriStand Inport){portnum=2, width=-1, stime=-1, dtype=auto, stype=auto, btype=1}
      mask prompts: portnum "Port number:"; width "Port dimensions (-1 for dynamically sized):"; stime "Sample time (-1 for inherited):"; dtype "Data type:"; stype "Signal type:"; btype "Block type:"
      mask help: Use this inport on any level of nested subsystems to allow NI VeriStand software to map signals to it.
      mask init:
      | NIVeriStandIO_init;
      settings: CopyFcn=NIVeriStand_MDL_functions('', 'IO_copy');  DeleteFcn=NIVeriStand_MDL_functions('', 'IO_delete');  MoveFcn=set_param(gcb, 'Mask', 'on');
      mask Callback portnum: NIVeriStand_MDL_functions('', 'IO_setportnum');
      mask TypeOptions dtype: auto | double | single | int8 | uint8 | int16 | uint16 | int32 | uint32 | boolean
      mask Callback dtype: NIVeriStand_MDL_functions('', 'IO_booleansignal');
      mask TypeOptions stype: auto | real | complex
      mask Display:
      | patch([-x x], [-y y], [.90980 .81960 .32156]);
      | plot([xrad -x x xrad], [yrad -y y yrad]);
      | fprintf('NI In%d', portnum);
  Out1 : Outport
  wires:
  RollRate/1 -> Rate Transition3/1
  YawRate/1 -> Rate Transition4/1
  Counter/1 -> Data Type Conversion11/1
  Bus Creator/1 -> Out1/1  "Checksums"
  MATLAB Function/1(RCM1_No_Cs) -> Data Type Conversion6/1  "RollYaw_Cs"
  MATLAB Function1/1(RCM2_No_Cs) -> Data Type Conversion5/1  "Accel_Cs"
  Accel_Counter/1 -> Data Type Conversion10/1
  LatAccel/1 -> Rate Transition/1
  LongAccel/1 -> Rate Transition1/1
  VertAccel/1 -> Rate Transition2/1
  VehRol_Qf/1 -> Data Type Conversion/1  "VehRol_Qf"
  VehYaw_Qf/1 -> Data Type Conversion1/1  "VehYaw_Qf"
  VehVert_Qf/1 -> Data Type Conversion4/1  "VehVert_Qf"
  VehLong_Qf/1 -> Data Type Conversion3/1  "VehLong_Qf"
  VehLat_Qf/1 -> Data Type Conversion2/1  "VehLat_Qf"
  Data Type Conversion/1 -> MATLAB Function/4(VehRolWActl_Qf), Bus Creator/2  "VehRol_Qf"
  Data Type Conversion1/1 -> Bus Creator/3, MATLAB Function/5(VehYawWActl_Qf)  "VehYaw_Qf"
  Data Type Conversion2/1 -> Bus Creator/5, MATLAB Function1/5(VehLatAActl_Qf)  "VehLat_Qf"
  Data Type Conversion3/1 -> Bus Creator/6, MATLAB Function1/6(VehLongAActl_Qf)  "VehLong_Qf"
  Data Type Conversion4/1 -> Bus Creator/7, MATLAB Function1/7(VehVertAActl_Qf)  "VehVert_Qf"
  Rate Transition3/1 -> MATLAB Function/2(VehRol_W_Actl)
  Rate Transition4/1 -> MATLAB Function/3(VehYaw_W_Actl)
  Rate Transition2/1 -> MATLAB Function1/4(VehVert2_A_Actl)
  Rate Transition1/1 -> MATLAB Function1/3(VehLong2_A_Actl)
  Rate Transition/1 -> MATLAB Function1/2(VehLat2_A_Actl)
  Data Type Conversion10/1 -> MATLAB Function1/1(VehLatLongVert_No_Cnt)
  Data Type Conversion11/1 -> MATLAB Function/1(VehRollYaw_No_Cnt)
  Data Type Conversion5/1 -> Bus Creator/4  "Accel_Cs"
  Data Type Conversion6/1 -> Bus Creator/1  "RollYaw_Cs"

== system P702_NI_SoftECU/SoftECU/RCM/Logic/Counters ==
  AccelCounter1 : S-Function  Priority=1  FunctionName=NIVeriStandIO  Parameters=width dtype portnum stime stype btype  SFunctionDeploymentMode=off  EnableBusSupport=off  mask(NI VeriStand Outport){portnum=1, width=-1, stime=-1, dtype=auto, stype=auto, btype=0}
      mask prompts: portnum "Port number:"; width "Port dimensions (-1 for dynamically sized):"; stime "Sample time (-1 for inherited):"; dtype "Data type:"; stype "Signal type:"; btype "Block type:"
      mask help: Use this outport on any level of nested subsystems to allow NI VeriStand software to map signals to it.
      mask init:
      | NIVeriStandIO_init;
      settings: CopyFcn=NIVeriStand_MDL_functions('', 'IO_copy');  DeleteFcn=NIVeriStand_MDL_functions('', 'IO_delete');  MoveFcn=set_param(gcb, 'Mask', 'on');
      mask Callback portnum: NIVeriStand_MDL_functions('', 'IO_setportnum');
      mask TypeOptions dtype: auto | double | single | int8 | uint8 | int16 | uint16 | int32 | uint32 | boolean
      mask Callback dtype: NIVeriStand_MDL_functions('', 'IO_booleansignal');
      mask TypeOptions stype: auto | real | complex
      mask Display:
      | patch([-x x], [-y y], [.90980 .81960 .32156]);
      | plot([xrad -x x xrad], [yrad -y y yrad]);
      | fprintf('NI Out%d', portnum);
  Bus Creator : BusCreator  Inputs=2
  Counter Limited : simulink/Sources/Counter Limited  uplimit=255  tsamp=.01
  Counter Limited1 : simulink/Sources/Counter Limited  uplimit=255  tsamp=.01
  Data Type Conversion : DataTypeConversion  OutDataTypeStr=uint8
  Data Type Conversion1 : DataTypeConversion  OutDataTypeStr=uint8
  Out1 : Outport
  wires:
  Counter Limited/1 -> Data Type Conversion/1
  Counter Limited1/1 -> Data Type Conversion1/1
  Bus Creator/1 -> Out1/1  "Counters"
  Data Type Conversion/1 -> Bus Creator/1  "RollYawCounter"
  Data Type Conversion1/1 -> AccelCounter1/1, Bus Creator/2  "AccelCounter"

== system P702_NI_SoftECU/SoftECU/RCM/Logic/StatusMessage ==
  note: Deployment Event = Threshold1Exceeded
      | Fuel Cutoff Event = Threshold2Exceeded
  note: RstrnImpactEvntStatus
      | 7 "Invalid"
      | 6 "Not_Used_4"
      | 5 "Threshold_2_Exceeded"
      | 4 "Not_Used_3"
      | 3 "Threshold_1_Exceeded"
      | 2 "Not_Used_2"
      | 1 "Not_Used_1"
      | 0 "Normal" ;
  In1 : Inport
  1-D Lookup Table : Lookup_n-D  NumberOfTableDimensions=1  BreakpointsForDimension1=[0 1 2]  Table=[0 3 5]  InterpMethod=Flat  RndMeth=Simplest  InputSameDT=on
  Constant : Constant  Value=0
  Terminator : Terminator
  Out1 : Outport
  wires:
  1-D Lookup Table/1 -> Out1/1  "RstrnImpactEvntStatus"
  In1/1 -> Terminator/1
  Constant/1 -> 1-D Lookup Table/1

== system P702_NI_SoftECU/SoftECU/RCM/Logic/UnitConversion ==
  In1 : Inport
  Bus Creator : BusCreator  Inputs=5
  Constant : Constant  Value=9.81
  Sum : Sum  Inputs=|++
  busselector1 : BusSelector  OutputSignals=RollRate_Veh_COG[deg/s],YawRate_Veh_COG[deg/s],a_x_veh_COG[m/s2],a_y_veh_COG[m/s2],a_z_Veh_COG[m/s2]
  deg to rad : Gain  Gain=pi/180
  deg to rad_ : Gain  Gain=pi/180
  deg to rad_1 : Gain
  deg to rad_2 : Gain
  deg to rad_3 : Gain
  Out1 : Outport
  wires:
  In1/1 -> busselector1/1
  deg to rad_/1 -> Bus Creator/1  "RollRate_Vehicle_CoG[rad|s]"
  deg to rad/1 -> Bus Creator/2  "YawRate_Vehicle_CoG[rad|s]"
  Bus Creator/1 -> Out1/1  "UnitConversion"
  deg to rad_1/1 -> Bus Creator/3  "a_x_Vehicle_CoG[m|s2]"
  deg to rad_2/1 -> Bus Creator/4  "a_y_Vehicle_CoG[m|s2]"
  deg to rad_3/1 -> Bus Creator/5  "a_z_Vehicle_CoG[m|s2]"
  busselector1/2 -> deg to rad/1  "<YawRate_Veh_COG[deg/s]>"
  busselector1/1 -> deg to rad_/1  "<RollRate_Veh_COG[deg/s]>"
  busselector1/3 -> deg to rad_1/1  "<a_x_veh_COG[m/s2]>"
  busselector1/4 -> deg to rad_2/1  "<a_y_veh_COG[m/s2]>"
  busselector1/5 -> Sum/1  "<a_z_Veh_COG[m/s2]>"
  Constant/1 -> Sum/2  "For Trial adding g (Serene )"
  Sum/1 -> deg to rad_3/1

== system P702_NI_SoftECU/SoftECU/RCM/Mapping/Accel_Data ==
  In1 : Inport
  Gain{,1..7} (8 alike) : Gain
  buscreator : BusCreator  Inputs=8
  busselector : BusSelector  OutputSignals=UnitConversion.a_y_Vehicle_CoG[m|s2],UnitConversion.a_x_Vehicle_CoG[m|s2],UnitConversion.a_z_Vehicle_CoG[m|s2],Counters.AccelCounter,Checksums.Accel_Cs,Checksums.VehLat_Qf,Checksums.VehLong_Qf,Checksums.VehVert_Qf
  Out1 : Outport
  wires:
  In1/1 -> busselector/1
  buscreator/1 -> Out1/1  "Accel_Data"
  Gain/1 -> buscreator/1  "VehLat2_A_Actl"
  Gain1/1 -> buscreator/2  "VehLong2_A_Actl"
  Gain2/1 -> buscreator/3  "VehVert2_A_Actl"
  busselector/3 -> Gain2/1  "<a_z_Vehicle_CoG[m|s2]>"
  busselector/1 -> Gain/1  "<a_y_Vehicle_CoG[m|s2]>"
  busselector/2 -> Gain1/1  "<a_x_Vehicle_CoG[m|s2]>"
  busselector/4 -> Gain3/1  "<AccelCounter>"
  busselector/5 -> Gain4/1  "<Accel_Cs>"
  Gain3/1 -> buscreator/4  "VehLatLongVert_No_Cnt"
  Gain4/1 -> buscreator/5  "VehLatLongVert_No_Cs"
  Gain6/1 -> buscreator/7  "VehLongAActl_D_Qf"
  busselector/7 -> Gain6/1  "<VehLong_Qf>"
  busselector/6 -> Gain5/1  "<VehLat_Qf>"
  Gain5/1 -> buscreator/6  "VehLatAActl_D_Qf"
  Gain7/1 -> buscreator/8  "VehVertAActl_D_Qf"
  busselector/8 -> Gain7/1  "<VehVert_Qf>"

== system P702_NI_SoftECU/SoftECU/RCM/Mapping/RCMStatusMessage2 ==
  In1 : Inport
  Constant : Constant
  Gain : Gain
  Gain1 : Gain
  buscreator : BusCreator  Inputs=2
  busselector : BusSelector  OutputSignals=RstrnImpactEvntStatus
  Out1 : Outport
  wires:
  busselector/1 -> Gain/1  "<RstrnImpactEvntStatus>"
  buscreator/1 -> Out1/1  "RCMStatusMessage2"
  In1/1 -> busselector/1
  Gain/1 -> buscreator/1  "RstrnImpactEvntStatus"
  Gain1/1 -> buscreator/2  "FirstRowBuckleDriver"
  Constant/1 -> Gain1/1

== system P702_NI_SoftECU/SoftECU/RCM/Mapping/Yaw_Data ==
  In1 : Inport
  Gain{,1..5} (6 alike) : Gain
  buscreator : BusCreator  Inputs=6
  busselector : BusSelector  OutputSignals=UnitConversion.RollRate_Vehicle_CoG[rad|s],UnitConversion.YawRate_Vehicle_CoG[rad|s],Counters.RollYawCounter,Checksums.RollYaw_Cs,Checksums.VehRol_Qf,Checksums.VehYaw_Qf
  Out1 : Outport
  wires:
  Gain/1 -> buscreator/1  "VehRol_W_Actl"
  buscreator/1 -> Out1/1  "Yaw_Data"
  In1/1 -> busselector/1
  Gain1/1 -> buscreator/2  "VehYaw_W_Actl"
  busselector/2 -> Gain1/1  "<YawRate_Vehicle_CoG[rad|s]>"
  busselector/1 -> Gain/1  "<RollRate_Vehicle_CoG[rad|s]>"
  Gain2/1 -> buscreator/3  "VehRollYaw_No_Cnt"
  Gain3/1 -> buscreator/4  "VehRollYawW_No_Cs"
  busselector/3 -> Gain2/1  "<RollYawCounter>"
  busselector/4 -> Gain3/1  "<RollYaw_Cs>"
  busselector/5 -> Gain4/1  "<VehRol_Qf>"
  busselector/6 -> Gain5/1  "<VehYaw_Qf>"
  Gain4/1 -> buscreator/5  "VehRolWActl_D_Qf"
  Gain5/1 -> buscreator/6  "VehYawWActl_D_Qf"

== system P702_NI_SoftECU/SoftECU/SCCM/Logic/Map_Inputs ==
  Reset[0|1] : Inport
  ECU_Commands[] : Inport  Port=2
  Maneuver : Subsystem
  Multiport Switch{1..8} (8 alike) : MultiPortSwitch  Inputs=2  SaturateOnIntegerOverflow=on
  Sw_ACC_BrakeMode[1Comfort|2AEBOnly|3AEBOff]1 : Constant
  Sw_ACC_Cancel[0Off|1On]1 : Constant  Value=0
  Sw_ACC_Control_Mode[1ManSched|2Manual] : Constant
  Sw_ACC_Off[0Off|1On]1 : Constant  Value=0
  Sw_ACC_On[0Off|1On]1 : Constant  Value=0
  Sw_ACC_Resume[0Off|1On]1 : Constant  Value=0
  Sw_ACC_Speed_Decrease[0Off|1On]1 : Constant  Value=0
  Sw_ACC_Speed_Increase[0Off|1On]1 : Constant  Value=0
  Sw_ACC_Speed_Set[0Off|1On]1 : Constant  Value=0
  Sw_ACC_On[0Off|1On] : Outport
  Sw_ACC_Off[0Off|1On] : Outport  Port=2
  Sw_ACC_Cancel[0Off|1On] : Outport  Port=3
  Sw_ACC_Resume[0Off|1On] : Outport  Port=4
  Sw_ACC_Speed_Set[0Off|1On] : Outport  Port=5
  Sw_ACC_Speed_Increase[0Off|1On] : Outport  Port=6
  Sw_ACC_Speed_Decrease[0Off|1On] : Outport  Port=7
  Sw_ACC_BrakeMode[1Comfort|2AEBOnly|3AEBOff] : Outport  Port=8
  wires:
  Maneuver/8(Sw_ACC_BrakeMode[1Comfort|2AEBOnly|3AEBOff]) -> Multiport Switch8/2
  Multiport Switch8/1 -> Sw_ACC_BrakeMode[1Comfort|2AEBOnly|3AEBOff]/1
  Reset[0|1]/1 -> Maneuver/2(Reset[0|1])
  Maneuver/7(Sw_ACC_Speed_Decrease[0Off|1On]) -> Multiport Switch1/2
  Maneuver/6(Sw_ACC_Speed_Increase[0Off|1On]) -> Multiport Switch2/2
  Maneuver/5(Sw_ACC_Speed_Set[0Off|1On]) -> Multiport Switch5/2
  Maneuver/4(Sw_ACC_Resume[0Off|1On]) -> Multiport Switch3/2
  Maneuver/3(Sw_ACC_Cancel[0Off|1On]) -> Multiport Switch4/2
  Maneuver/2(Sw_ACC_Off[0Off|1On]) -> Multiport Switch6/2
  ECU_Commands[]/1 -> Maneuver/1(ECU_Commands[])
  Multiport Switch1/1 -> Sw_ACC_Speed_Decrease[0Off|1On]/1
  Multiport Switch2/1 -> Sw_ACC_Speed_Increase[0Off|1On]/1
  Multiport Switch5/1 -> Sw_ACC_Speed_Set[0Off|1On]/1
  Multiport Switch3/1 -> Sw_ACC_Resume[0Off|1On]/1
  Multiport Switch4/1 -> Sw_ACC_Cancel[0Off|1On]/1
  Multiport Switch6/1 -> Sw_ACC_Off[0Off|1On]/1
  Multiport Switch7/1 -> Sw_ACC_On[0Off|1On]/1
  Sw_ACC_Control_Mode[1ManSched|2Manual]/1 -> Multiport Switch1/1, Multiport Switch8/1, Multiport Switch2/1, Multiport Switch5/1, Multiport Switch3/1, Multiport Switch4/1, Multiport Switch6/1, Multiport Switch7/1  "Sw_ACC_Control_Mode[1ManSched|2Manual]"
  Sw_ACC_On[0Off|1On]1/1 -> Multiport Switch7/3  "Sw_ACC_On[Off|1On]"
  Sw_ACC_Off[0Off|1On]1/1 -> Multiport Switch6/3  "Sw_ACC_Off[0Off|1On]"
  Sw_ACC_Cancel[0Off|1On]1/1 -> Multiport Switch4/3  "Sw_ACC_Cancel[0Off|1On]"
  Sw_ACC_Resume[0Off|1On]1/1 -> Multiport Switch3/3  "Sw_ACC_Resume[0Off|1On]"
  Sw_ACC_Speed_Set[0Off|1On]1/1 -> Multiport Switch5/3  "Sw_ACC_Speed_Set[0Off|1On]"
  Sw_ACC_Speed_Increase[0Off|1On]1/1 -> Multiport Switch2/3  "Sw_ACC_Speed_Increase[0Off|1On]"
  Sw_ACC_Speed_Decrease[0Off|1On]1/1 -> Multiport Switch1/3  "Sw_ACC_Speed_Decrease[0Off|1On]"
  Sw_ACC_BrakeMode[1Comfort|2AEBOnly|3AEBOff]1/1 -> Multiport Switch8/3  "Sw_ACC_BrakeMode[1Comfort|2AEBOnly|3AEBOff]"
  Maneuver/1(Sw_ACC_On[0Off|1On]) -> Multiport Switch7/2
